simulink model "chap8_8sim"  (R2015a)
settings: Solver=ode45  StartTime=0.0  StopTime=100  RelTol=1e-3
settings Model: Creator=zhr  LastModifiedBy=zhr

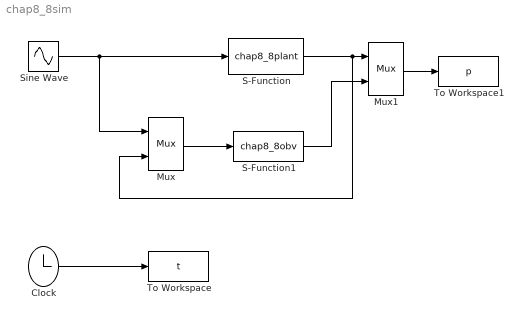
== system chap8_8sim ==
  Clock : Clock
  Mux : Mux  Inputs=2
  Mux1 : Mux  Inputs=2
  S-Function : S-Function  FunctionName=chap8_8plant
  S-Function1 : S-Function  FunctionName=chap8_8obv
  Sine Wave : Sin  Amplitude=150  Frequency=0.1  SampleTime=0
  To Workspace : ToWorkspace  VariableName=t  SampleTime=-1
  To Workspace1 : ToWorkspace  VariableName=p  SampleTime=-1
  wires:
  Clock/1 -> To Workspace/1
  Sine Wave/1 -> Mux/1, S-Function/1
  Mux/1 -> S-Function1/1
  S-Function1/1 -> Mux1/2
  S-Function/1 -> Mux/2, Mux1/1
  Mux1/1 -> To Workspace1/1
